simulink model "diff1"  (R2018a)
settings: Solver=VariableStepAuto  StartTime=0.0  StopTime=10.0  RelTol=1e-3
model workspace: external: MAT-File params.mat (data not in the file)
settings Model: Creator=fangxz  LastModifiedBy=fangxz

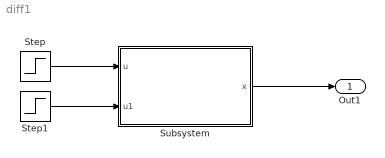
== system diff1 ==
  Step : Step  SampleTime=0
  Step1 : Step  After=0.1  SampleTime=0
  Subsystem : Subsystem
  Out1 : Outport
  wires:
  Subsystem/1(x) -> Out1/1
  Step1/1 -> Subsystem/2(u1)
  Step/1 -> Subsystem/1(u)

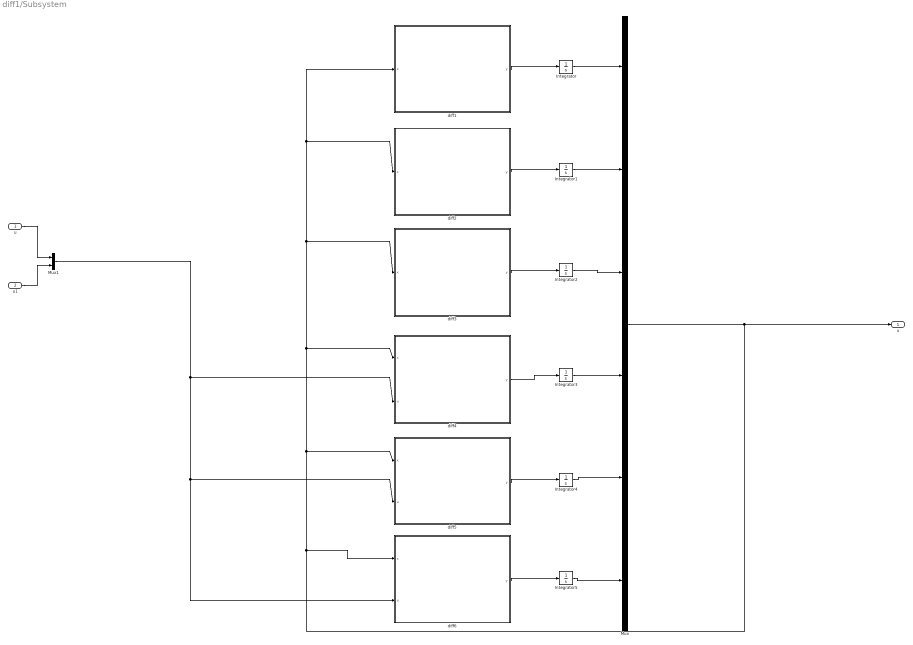
== system diff1/Subsystem ==
  u : Inport
  u1 : Inport  Port=2
  Integrator{,1..5} (6 alike) : Integrator
  Mux : Mux  Inputs=6
  Mux1 : Mux  Inputs=2
  diff1 : MATLAB Function  TreatAsAtomicUnit=on
  diff2 : MATLAB Function  TreatAsAtomicUnit=on
  diff3 : MATLAB Function  TreatAsAtomicUnit=on
  diff4 : MATLAB Function  TreatAsAtomicUnit=on
  diff5 : MATLAB Function  TreatAsAtomicUnit=on
  diff6 : MATLAB Function  TreatAsAtomicUnit=on
  x : Outport
  wires:
  diff1/1(y) -> Integrator/1
  diff2/1(y) -> Integrator1/1
  diff3/1(y) -> Integrator2/1
  diff4/1(y) -> Integrator3/1
  diff5/1(y) -> Integrator4/1
  diff6/1(y) -> Integrator5/1
  Mux/1 -> diff6/1(x), diff4/1(x), diff2/1(x), diff1/1(x), diff3/1(x), diff5/1(x), x/1
  Mux1/1 -> diff6/2(u), diff5/2(u), diff4/2(u)
  Integrator/1 -> Mux/1
  Integrator1/1 -> Mux/2
  Integrator2/1 -> Mux/3
  Integrator3/1 -> Mux/4
  Integrator4/1 -> Mux/5
  Integrator5/1 -> Mux/6
  u1/1 -> Mux1/2
  u/1 -> Mux1/1

== matlab function diff1/Subsystem/diff2 ==
  data: x input; y output
function y = diff2(x)
y =  x(4)*sin(x(3))+x(5)*cos(x(3));

== matlab function diff1/Subsystem/diff1 ==
  data: x input; y output
function y = diff1(x)
y= x(4)*cos(x(3))-x(5)*sin(x(3));

== matlab function diff1/Subsystem/diff3 ==
  data: x input; y output
function y = fcn(x)
y = x(6);

== matlab function diff1/Subsystem/diff4 ==
  data: x input; u input; y output
function y = fcn(x,u)
m = 1573;
Iz = 2873;
l_f = 1.35;
l_r = 1.35;
W_f=l_r/(l_f+l_r);
W_r=l_f/(l_f+l_r);
Cm1=17303;
Cm2=175;
Cr0=120;
Cr2=0.5*1.225*0.35*2.5;
B_r = 13;
C_r = 2;
D_r = W_f*m*9.81*1.2;
B_f = 13;
C_f = 2;
D_f = W_r*m*9.81*1.2;
y =  1/m*((Cm1*u(2)-Cm2*u(2)*x(4)-Cr0-Cr2*x(4)^2) - (D_f*sin(C_f*atan(B_f*( -atan2(l_f*x(6) + x(5),x(4))+u(1)))))*sin(u(1)) + m*x(5)*x(6));

== matlab function diff1/Subsystem/diff5 ==
  data: x input; u input; y output
function y = fcn(x,u)
m = 1573;
Iz = 2873;
l_f = 1.35;
l_r = 1.35;
W_f=l_r/(l_f+l_r);
W_r=l_f/(l_f+l_r);
Cm1=17303;
Cm2=175;
Cr0=120;
Cr2=0.5*1.225*0.35*2.5;
B_r = 13;
C_r = 2;
D_r = W_f*m*9.81*1.2;
B_f = 13;
C_f = 2;
D_f = W_r*m*9.81*1.2;
y = 1/m*(D_r*sin(C_r*atan(B_r*(atan2(l_r*x(6) - x(5),x(4))))) + (D_f*sin(C_f*atan(B_f*( -atan2(l_f*x(6) + x(5),x(4))+u(1)))))*cos(u(1)) - m*x(4)*x(6));

== matlab function diff1/Subsystem/diff6 ==
  data: x input; u input; y output
function y = fcn(x,u)
m = 1573;
Iz = 2873;
l_f = 1.35;
l_r = 1.35;
W_f=l_r/(l_f+l_r);
W_r=l_f/(l_f+l_r);
Cm1=17303;
Cm2=175;
Cr0=120;
Cr2=0.5*1.225*0.35*2.5;
B_r = 13;
C_r = 2;
D_r = W_f*m*9.81*1.2;
B_f = 13;
C_f = 2;
D_f = W_r*m*9.81*1.2;
y =  1/Iz*((D_f*sin(C_f*atan(B_f*( -atan2(l_f*x(6) + x(5),x(4))+u(1)))))*l_f*cos(u(1))- (D_r*sin(C_r*atan(B_r*(atan2(l_r*x(6) - x(5),x(4))))))*l_r)
